simulink model "verify_HX_finned_tube_mdl"  (R2016b)
settings: Solver=VariableStepDiscrete  StartTime=0  StopTime=10  MaxStep=1  RelTol=1e-3  EnableMultiTasking=on
InitFcn:
  | height =1.47;
  | dia = 0.525;
  | nodes = 5;
libraries: carnot x3, simulink x1
settings Model: Creator=drhf  LastModifiedBy=drhf
settings DataIOCC: SaveFormat=Array  SignalLoggingSaveFormat=ModelDataLogs
settings OptimizationCC: ExpressionDepthLimit=2147483647  LifeSpan=inf
settings DebuggingCC: UnderspecifiedInitializationDetection=Classic  MergeDetectMultiDrivingBlocksExec=none  SolverPrmCheckMsg=warning  FcnCallInpInsideContextMsg=warning  StateNameClashWarn=warning  SFUnexpectedBacktrackingDiag=warning  SFNoUnconditionalDefaultTransitionDiag=warning  SFExecutionAtInitializationDiag=none
settings HardwareCC: ProdBitPerPointer=32  ProdBitPerSizeT=32  ProdBitPerPtrDiffT=32  ProdLargestAtomicFloat=None  ProdIntDivRoundTo=Undefined  ProdEndianess=Unspecified  ProdWordSize=32  ProdHWDeviceType=32-bit Generic
settings ModelReferenceCC: PropagateSignalLabelsOutOfModel=off
settings GRTTargetCC: TargetLangStandard=C89/C90 (ANSI)  GeneratePreprocessorConditionals=Disable all  CombineOutputUpdateFcns=off  GRTInterface=on
settings ConfigComp: CovMetricSettings=dw  CovHtmlReporting=on  CovSaveCumulativeToWorkspaceVar=on  CovSaveSingleToWorkspaceVar=on  CovExternalEMLEnable=off

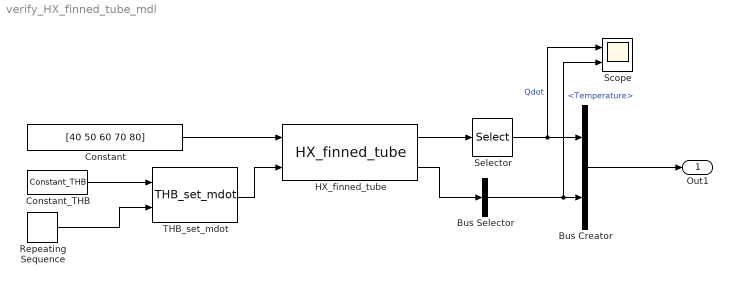
== system verify_HX_finned_tube_mdl ==
  Bus Creator : BusCreator  Inputs=2
  Bus Selector : BusSelector  OutputSignals=Temperature
  Constant : Constant  Value=[40 50 60 70 80]
  Constant_THB : carnot/Source/Simple/Constant_THB  t=90  mdot=500/3600  p=1e5  mID=No Pressure Drop  fluid=Water  mix=0  mix2=0  mix3=0  dia=0.02  hgt=0
  HX_finned_tube : carnot/Storage/Thermal/Storage_Ports/HX_finned_tube  h_in=0.9  h_out=0.1  hgt=1  dpipe=0.03  swall=0.001  lpipe=10  cond=50  dfin=0.05  sfin=0.002  nfin=100  height=-0.8  dplin=100  dpqua=100  nodes=5
  Repeating Sequence : simulink/Sources/Repeating Sequence  rep_seq_t=[0 5 10]  rep_seq_y=[100/3600 500/3600 100/3600]
  Scope : Scope  NumInputPorts=2
  Selector : Selector  InputPortWidth=28  IndexOptions=Index vector (dialog)  Indices=[21:25]  OutputSizes=1
  THB_set_mdot : carnot/Source/Simple/THB_set_mdot
  Out1 : Outport
  wires:
  HX_finned_tube/1 -> Selector/1
  HX_finned_tube/2 -> Bus Selector/1
  Selector/1 -> Scope/1, Bus Creator/1  "Qdot"
  Bus Selector/1 -> Scope/2, Bus Creator/2  "<Temperature>"
  Bus Creator/1 -> Out1/1
  Constant/1 -> HX_finned_tube/1
  THB_set_mdot/1 -> HX_finned_tube/2
  Constant_THB/1 -> THB_set_mdot/1
  Repeating Sequence/1 -> THB_set_mdot/2
